simulink model "task5_5_e"  (R2015a)
settings: Solver=ode45  StartTime=0.0  StopTime=sim_t  RelTol=1e-3
undefined symbols (not defined in the file): K_pd, PSI_r, T_d, T_f, T_s
libraries: simulink x2
settings Model: Creator=markh  LastModifiedBy=perakj
settings DataIOCC: SignalLoggingSaveFormat=ModelDataLogs  SignalLoggingName=sigsOut
settings OptimizationCC: InitFltsAndDblsToZero=on
settings DebuggingCC: SaveWithParameterizedLinksMsg=none  UnderspecifiedInitializationDetection=Classic  MergeDetectMultiDrivingBlocksExec=none  SignalResolutionControl=TryResolveAllWithWarning  MultiTaskDSMMsg=warning  MultiTaskCondExecSysMsg=none  FcnCallInpInsideContextMsg=UseLocalSettings  StateNameClashWarn=warning
settings HardwareCC: TargetUnknown=on
settings GRTTargetCC: TargetFcnLib=ansi_tfl_tmw.mat  CombineOutputUpdateFcns=off  GRTInterface=on

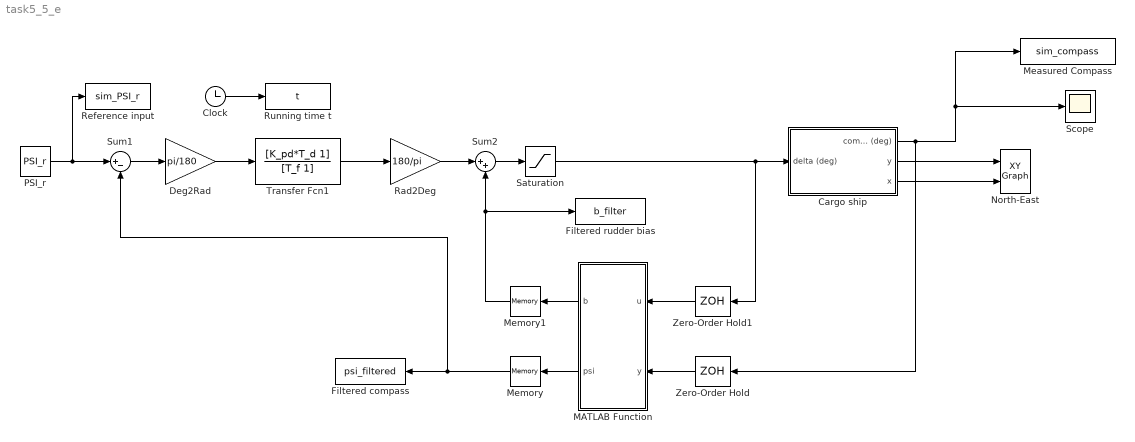
== system task5_5_e ==
  Cargo ship : Subsystem  mask(Simple shipmodel for a cargo ship){noise=on, current=on, logic=on}
      mask prompts: noise "measurement noise"; logic "waves"
      mask help:
      | Measurement noise:
      | 	checked = noise on
      | 	unchecked = noise off
      |
      | Current:
      | 	checked = current on
      | 	unchecked = current off
      |
      | Waves:
      | 	checked = waves on
      | 	unchecked = waves off
      |
      | Author: Jørgen Spjøtvold, 9/10-2003
      | TTK 4115 Linear system theory.
      | Modified by Jostein Bakkeheim 26/10-2006
  Clock : Clock
  Deg2Rad : Gain  Gain=pi/180
  Filtered compass : ToWorkspace  VariableName=psi_filtered  SampleTime=-1
  Filtered rudder bias : ToWorkspace  VariableName=b_filter  SampleTime=-1
  MATLAB Function : MATLAB Function  TreatAsAtomicUnit=on
  Measured Compass : ToWorkspace  VariableName=sim_compass  SampleTime=-1
  Memory : Memory
  Memory1 : Memory
  North-East : simulink/Sinks/XY Graph  xmin=-5000  xmax=5000  ymin=-5000  ymax=5000  st=-1
  PSI_r : Constant  Value=PSI_r
  Rad2Deg : Gain  Gain=180/pi
  Reference input : ToWorkspace  VariableName=sim_PSI_r  SampleTime=-1
  Running time t : ToWorkspace  VariableName=t  SampleTime=-1
  Saturation : Saturate  UpperLimit=35  LowerLimit=-35
  Scope : Scope
      settings: ShowLegends=on  YMin=-0.25  YMax=4.75  SaveName=PD_simulink
  Sum1 : Sum  Inputs=|+-
  Sum2 : Sum  Inputs=|++
  Transfer Fcn1 : TransferFcn  Numerator=[K_pd*T_d 1]  Denominator=[T_f 1]
  Zero-Order Hold : ZeroOrderHold  SampleTime=T_s
  Zero-Order Hold1 : ZeroOrderHold  SampleTime=T_s
  wires:
  Cargo ship/3(x) -> North-East/2
  Cargo ship/2(y) -> North-East/1
  Cargo ship/1(compass (deg)) -> Zero-Order Hold/1, Measured Compass/1, Scope/1
  Deg2Rad/1 -> Transfer Fcn1/1
  Transfer Fcn1/1 -> Rad2Deg/1
  PSI_r/1 -> Sum1/1, Reference input/1
  Sum1/1 -> Deg2Rad/1
  Clock/1 -> Running time t/1
  Saturation/1 -> Zero-Order Hold1/1, Cargo ship/1(delta (deg))
  Zero-Order Hold/1 -> MATLAB Function/2(y)
  Zero-Order Hold1/1 -> MATLAB Function/1(u)
  MATLAB Function/2(psi) -> Memory/1
  MATLAB Function/1(b) -> Memory1/1
  Memory1/1 -> Sum2/2, Filtered rudder bias/1
  Rad2Deg/1 -> Sum2/1
  Sum2/1 -> Saturation/1
  Memory/1 -> Filtered compass/1, Sum1/2

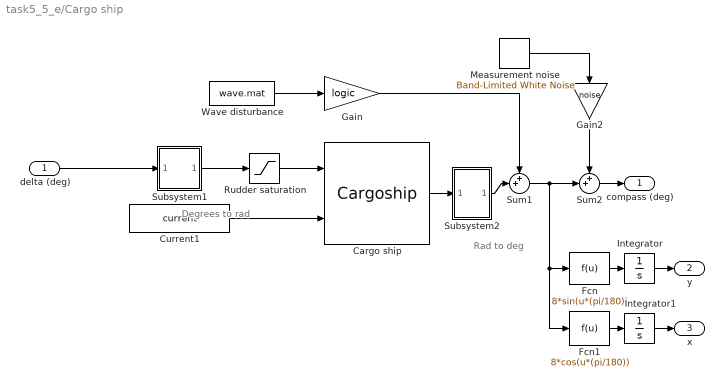
== system task5_5_e/Cargo ship ==
  note: Degrees to rad
  note: Rad to deg
  delta (deg) : Inport
  Cargo ship : S-Function  FunctionName=Cargoship  mask(Cargo ship){}
      mask help:
      | S-function which simulates a cargo ship.
      |
      | Author: Jørgen Spjøtvold
      | 20.10-2003
      | Modified by Jostein Bakkeheim 27.10.2006
  Current1 : Constant  Value=current
  Fcn : Fcn  Expr=8*sin(u*(pi/180))
  Fcn1 : Fcn  Expr=8*cos(u*(pi/180))
  Gain : Gain  Gain=logic  SaturateOnIntegerOverflow=on  OutDataTypeStr=Inherit: Same as input  ParamDataTypeStr=Inherit: Same as input
  Gain2 : Gain  Gain=noise  SaturateOnIntegerOverflow=on  OutDataTypeStr=Inherit: Same as input  ParamDataTypeStr=Inherit: Same as input
  Integrator : Integrator
  Integrator1 : Integrator
  Measurement noise : simulink/Sources/Band-Limited White Noise  Cov=[0.001]  Ts=.5  seed=[23341]
  Rudder saturation : Saturate  UpperLimit=45*(pi/180)  LowerLimit=-45*(pi/180)
  Subsystem1 : Subsystem  mask(degrees to radians){}
      mask help: Converts degrees to radians
      mask Display: fprintf('D2R');
  Subsystem2 : Subsystem  mask(radians to degrees){}
      mask help: Converts radians to degrees
      mask Display: fprintf('R2D');
  Sum1 : Sum  Inputs=++|  SaturateOnIntegerOverflow=on
  Sum2 : Sum  Inputs=++|  SaturateOnIntegerOverflow=on
  Wave disturbance : FromFile  FileName=wave.mat  SampleTime=0
  compass (deg) : Outport
  y : Outport  Port=2
  x : Outport  Port=3
  wires:
  delta (deg)/1 -> Subsystem1/1(In1)
  Fcn/1 -> Integrator/1
  Integrator/1 -> y/1
  Fcn1/1 -> Integrator1/1
  Integrator1/1 -> x/1
  Wave disturbance/1 -> Gain/1
  Subsystem2/1(Out1) -> Sum1/2
  Gain/1 -> Sum1/1
  Sum1/1 -> Fcn/1, Fcn1/1, Sum2/2
  Cargo ship/1 -> Subsystem2/1(In1)
  Subsystem1/1(Out1) -> Rudder saturation/1
  Rudder saturation/1 -> Cargo ship/1
  Sum2/1 -> compass (deg)/1
  Measurement noise/1 -> Gain2/1
  Gain2/1 -> Sum2/1
  Current1/1 -> Cargo ship/2

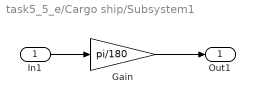
== system task5_5_e/Cargo ship/Subsystem1 ==
  In1 : Inport
  Gain : Gain  Gain=pi/180  SaturateOnIntegerOverflow=on  OutDataTypeStr=Inherit: Same as input  ParamDataTypeStr=Inherit: Same as input
  Out1 : Outport
  wires:
  Gain/1 -> Out1/1
  In1/1 -> Gain/1

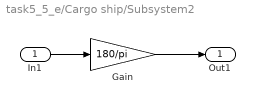
== system task5_5_e/Cargo ship/Subsystem2 ==
  In1 : Inport
  Gain : Gain  Gain=180/pi  SaturateOnIntegerOverflow=on  OutDataTypeStr=Inherit: Same as input  ParamDataTypeStr=Inherit: Same as input
  Out1 : Outport
  wires:
  Gain/1 -> Out1/1
  In1/1 -> Gain/1

== matlab function task5_5_e/MATLAB Function ==
  data: u input; b output size=1; y input; psi output size=1; data parameter
function [b,psi] = fcn(u, y, data)
%#codegen
persistent init_flag A B C E Q R P_ x_ I 

if (isempty(init_flag))
    init_flag = 1;
    
    % Initialization for system
    [A,B,C,E,Q,R,P_,x_, I] = deal(data.Ad,data.Bd,data.Cd,data.Ed,data.Q, ...
                                data.R, data.P_0, data.X_0, data.I);
end
x = zeros(5,1);
P = zeros(5,5);

% 1 - Compute the Kalman Gain
L = P_*C'*inv((C*P_*C'+R));
% 2 - Update estimate with measurment
x = x_ + L*(y-C*x_);
% 3 - Update error covariance matrix
P = (I - L*C)*P_*(I-L*C)'+L*R*L';
% 4 - Projet ahead
x_ = A*x + B*u;
P_ = A*P*A' + E*Q*E';

psi = x(3); b = x(5);
